simulink model "untitled"  (R2014a)
settings: Solver=ode45  StartTime=0.0  StopTime=10.0  RelTol=1e-3
undefined symbols (not defined in the file or in its folder): sigbuilder_block
libraries: simulink x4
settings Model: Creator=Dell  LastModifiedBy=Dell

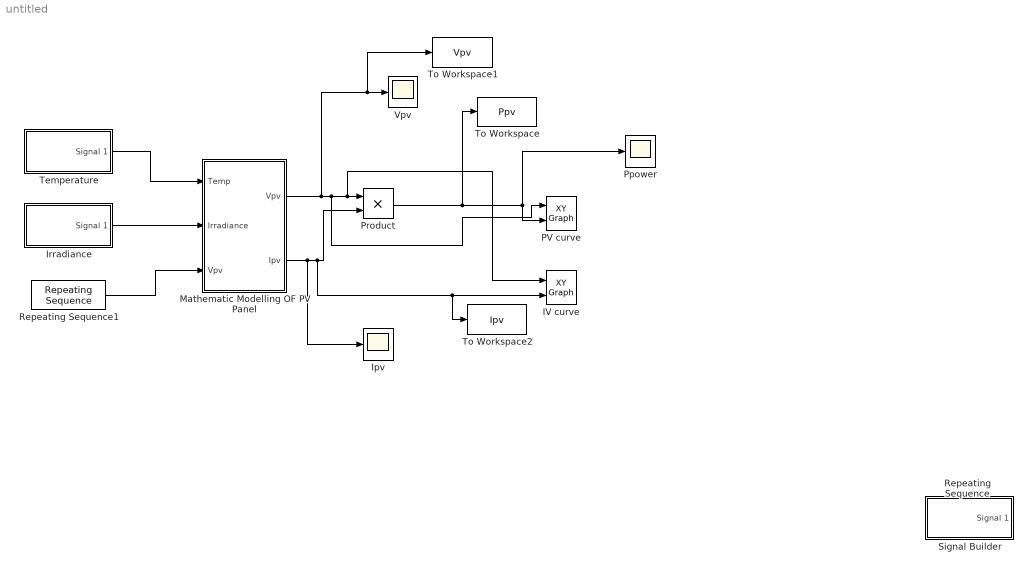
== system untitled ==
  IV curve : simulink/Sinks/XY Graph  xmin=-1  xmax=1  ymin=-1  ymax=1  st=-1
  Ipv : Scope
  Irradiance : Subsystem  Tag=STV Subsys  LoadFcn=sigbuilder_block('load');  StartFcn=sigbuilder_block('start');  StopFcn=sigbuilder_block('stop');  ClipboardFcn=sigbuilder_block('clipboard');  mask(Sigbuilder block){}
      mask help: Simulink:masks:SigbuilderBlock_MD
      mask init:
      | if ~strcmp(get_param(bdroot(gcbh),'SimulationStatus'),'stopped') tuvar = sigbuilder_block('maskInit'); end
      settings: CopyFcn=sigbuilder_block('copy');  DeleteFcn=sigbuilder_block('delete');  ModelCloseFcn=sigbuilder_block('modelClose');  PreSaveFcn=sigbuilder_block('preSave');  PauseFcn=sigbuilder_block('pause');  ContinueFcn=sigbuilder_block('continue');  NameChangeFcn=sigbuilder_block('namechange');  OpenFcn=sigbuilder_block('open',[441 189.75 543 385.5 ]);  CloseFcn=sigbuilder_block('close');
      mask Display: plot(0, 0, 100, 100,[2, 2, 32, 32, 2], [68, 8, 8, 68, 68],[32, 2], [38, 38], [32, 19, 2],[53, 60, 44], [32, 17, 17, 2],[16, 16, 31, 31]);txt = getActiveGroup(gcbh);text(2, 100, txt,'verticalAlignment', 'top');
  Mathematic Modelling OF PV Panel : Subsystem
  PV curve : simulink/Sinks/XY Graph  xmin=-1  xmax=1  ymin=-1  ymax=1  st=-1
  "Ppower " : Scope
      settings: SaveName=ScopeData2
  Product : Product
  Repeating Sequence : simulink/Sources/Repeating Sequence  rep_seq_t=[0 2]  rep_seq_y=[0 2]
  Repeating Sequence1 : simulink/Sources/Repeating Sequence  rep_seq_t=[0 2]  rep_seq_y=[0 2]
  Signal Builder : Subsystem  Tag=STV Subsys  LoadFcn=sigbuilder_block('load');  StartFcn=sigbuilder_block('start');  StopFcn=sigbuilder_block('stop');  ClipboardFcn=sigbuilder_block('clipboard');  mask(Sigbuilder block){}
      mask help: Simulink:masks:SigbuilderBlock_MD
      mask init:
      | if ~strcmp(get_param(bdroot(gcbh),'SimulationStatus'),'stopped') tuvar = sigbuilder_block('maskInit'); end
      settings: CopyFcn=sigbuilder_block('copy');  DeleteFcn=sigbuilder_block('delete');  ModelCloseFcn=sigbuilder_block('modelClose');  PreSaveFcn=sigbuilder_block('preSave');  PauseFcn=sigbuilder_block('pause');  ContinueFcn=sigbuilder_block('continue');  NameChangeFcn=sigbuilder_block('namechange');  OpenFcn=sigbuilder_block('open',[437.6 199.2 550.4 400 ]);  CloseFcn=sigbuilder_block('close');
      mask Display: plot(0, 0, 100, 100,[2, 2, 32, 32, 2], [68, 8, 8, 68, 68],[32, 2], [38, 38], [32, 19, 2],[53, 60, 44], [32, 17, 17, 2],[16, 16, 31, 31]);txt = getActiveGroup(gcbh);text(2, 100, txt,'verticalAlignment', 'top');
  "Temperature " : Subsystem  Tag=STV Subsys  LoadFcn=sigbuilder_block('load');  StartFcn=sigbuilder_block('start');  StopFcn=sigbuilder_block('stop');  ClipboardFcn=sigbuilder_block('clipboard');  mask(Sigbuilder block){}
      mask help: Simulink:masks:SigbuilderBlock_MD
      mask init:
      | if ~strcmp(get_param(bdroot(gcbh),'SimulationStatus'),'stopped') tuvar = sigbuilder_block('maskInit'); end
      settings: CopyFcn=sigbuilder_block('copy');  DeleteFcn=sigbuilder_block('delete');  ModelCloseFcn=sigbuilder_block('modelClose');  PreSaveFcn=sigbuilder_block('preSave');  PauseFcn=sigbuilder_block('pause');  ContinueFcn=sigbuilder_block('continue');  NameChangeFcn=sigbuilder_block('namechange');  OpenFcn=sigbuilder_block('open',[351 -51.75 543 385.5 ]);  CloseFcn=sigbuilder_block('close');
      mask Display: plot(0, 0, 100, 100,[2, 2, 32, 32, 2], [68, 8, 8, 68, 68],[32, 2], [38, 38], [32, 19, 2],[53, 60, 44], [32, 17, 17, 2],[16, 16, 31, 31]);txt = getActiveGroup(gcbh);text(2, 100, txt,'verticalAlignment', 'top');
  To Workspace : ToWorkspace  VariableName=Ppv  SaveFormat=Timeseries  SampleTime=-1
  To Workspace1 : ToWorkspace  VariableName=Vpv  SaveFormat=Timeseries  SampleTime=-1
  To Workspace2 : ToWorkspace  VariableName=Ipv  SaveFormat=Timeseries  SampleTime=-1
  Vpv : Scope
  wires:
  Mathematic Modelling OF PV Panel/2(Ipv) -> Ipv/1, To Workspace2/1, IV curve/2, Product/2
  Mathematic Modelling OF PV Panel/1("Vpv ") -> To Workspace1/1, Vpv/1, PV curve/1, IV curve/1, Product/1
  Product/1 -> To Workspace/1, PV curve/2, "Ppower "/1
  "Temperature "/1(Signal 1) -> Mathematic Modelling OF PV Panel/1(Temp)
  Irradiance/1(Signal 1) -> Mathematic Modelling OF PV Panel/2(Irradiance)
  Repeating Sequence1/1 -> Mathematic Modelling OF PV Panel/3(Vpv)

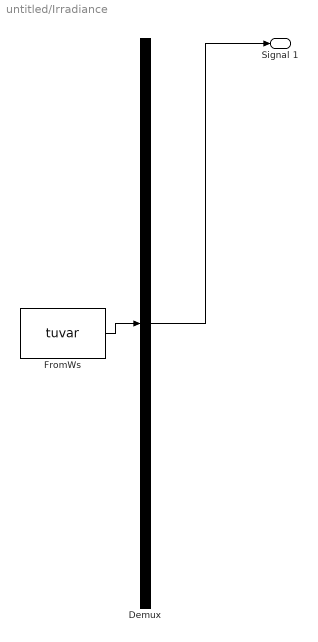
== system untitled/Irradiance ==
  Demux : Demux  Tag=STV Demux  Outputs=1
  FromWs : FromWorkspace  Tag=STV FromWs  VariableName=tuvar  SampleTime=0
      SigBuilderData=|
      | common.afterFinalStr = 'Extrapolate'
      | common.sampleTime = 0
      | dataSet.timeRange = [0 10]
      | dataSet.name = 'Group 1'
      | sbobj.Groups.Name = 'Group 1'
      | sbobj.Groups.Signals.Name = 'Signal 1'
      | sbobj.Groups.Signals.XData = [0 4 4 6 6 10]
      | sbobj.Groups.Signals.YData = [0 0 1 1 0 0]
  Signal 1 : Outport  Tag=STV Outport
  wires:
  Demux/1 -> Signal 1/1
  FromWs/1 -> Demux/1

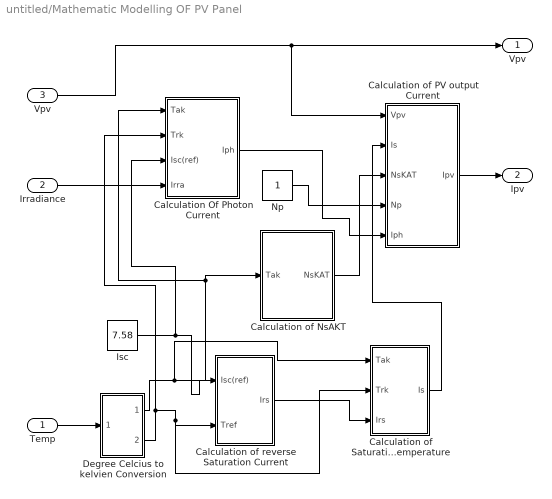
== system untitled/Mathematic Modelling OF PV Panel ==
  Temp : Inport
  Irradiance : Inport  Port=2
  Vpv : Inport  Port=3
  "Calculation Of Photon Current " : Subsystem
  Calculation of Saturation Current Varies With Temperature : Subsystem
  Calculation of NsAKT : Subsystem
  "Calculation of PV output Current " : Subsystem
  Calculation of reverse Saturation Current : Subsystem
  Degree Celcius to kelvien Conversion : Subsystem
  Isc : Constant  Value=7.58
  Np : Constant
  "Vpv " : Outport
  Ipv : Outport  Port=2
  wires:
  Calculation of Saturation Current Varies With Temperature/1(Is) -> "Calculation of PV output Current "/2(Is)
  Calculation of reverse Saturation Current/1(Irs) -> Calculation of Saturation Current Varies With Temperature/3("Irs ")
  Np/1 -> "Calculation of PV output Current "/4(Np)
  Temp/1 -> Degree Celcius to kelvien Conversion/1("Top ")
  "Calculation of PV output Current "/1("Ipv ") -> Ipv/1
  Irradiance/1 -> "Calculation Of Photon Current "/4(Irra)
  Degree Celcius to kelvien Conversion/1(Tak) -> Calculation of Saturation Current Varies With Temperature/1(Tak), "Calculation Of Photon Current "/1(Tak), Calculation of NsAKT/1("Tak ")
  "Calculation Of Photon Current "/1(Iph) -> "Calculation of PV output Current "/5(Iph)
  Calculation of NsAKT/1(NsKAT) -> "Calculation of PV output Current "/3(NsKAT)
  Isc/1 -> "Calculation Of Photon Current "/3(Isc(ref)), Calculation of reverse Saturation Current/1("Isc(ref) ")
  Degree Celcius to kelvien Conversion/2(Trk) -> "Calculation Of Photon Current "/2(Trk), Calculation of Saturation Current Varies With Temperature/2("Trk "), Calculation of reverse Saturation Current/2("Tref ")
  Vpv/1 -> "Vpv "/1, "Calculation of PV output Current "/1(Vpv)

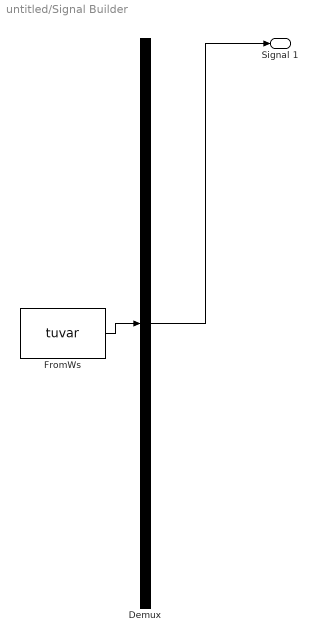
== system untitled/Signal Builder ==
  Demux : Demux  Tag=STV Demux  Outputs=1
  FromWs : FromWorkspace  Tag=STV FromWs  VariableName=tuvar  SampleTime=0
      SigBuilderData=|
      | common.afterFinalStr = 'Extrapolate'
      | common.sampleTime = 0
      | dataSet.timeRange = [0 10]
      | dataSet.name = 'Group 1'
      | sbobj.Groups.Name = 'Group 1'
      | sbobj.Groups.Signals.Name = 'Signal 1'
      | sbobj.Groups.Signals.XData = [0 4 4 6 6 10]
      | sbobj.Groups.Signals.YData = [0 0 1 1 0 0]
  Signal 1 : Outport  Tag=STV Outport
  wires:
  Demux/1 -> Signal 1/1
  FromWs/1 -> Demux/1

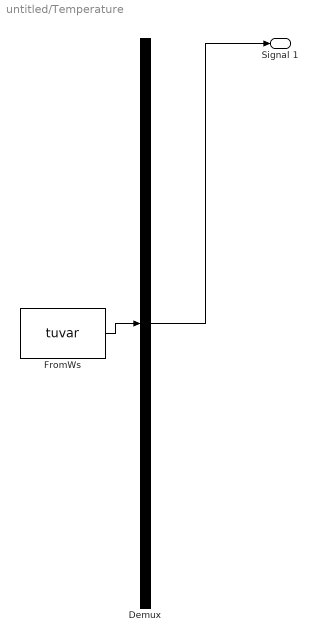
== system untitled/Temperature  ==
  Demux : Demux  Tag=STV Demux  Outputs=1
  FromWs : FromWorkspace  Tag=STV FromWs  VariableName=tuvar  SampleTime=0
      SigBuilderData=|
      | common.afterFinalStr = 'Extrapolate'
      | common.sampleTime = 0
      | dataSet.timeRange = [0 10]
      | dataSet.name = 'Group 1'
      | sbobj.Groups.Name = 'Group 1'
      | sbobj.Groups.Signals.Name = 'Signal 1'
      | sbobj.Groups.Signals.XData = [0 1 1 2 2 10]
      | sbobj.Groups.Signals.YData = [25 25 50 50 75 75]
  Signal 1 : Outport  Tag=STV Outport
  wires:
  FromWs/1 -> Demux/1
  Demux/1 -> Signal 1/1

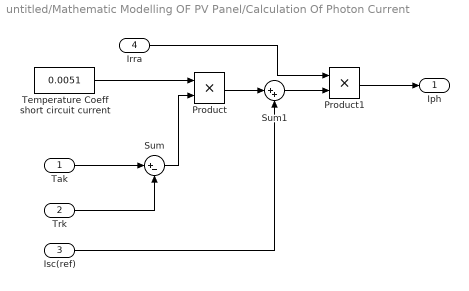
== system untitled/Mathematic Modelling OF PV Panel/Calculation Of Photon Current  ==
  Tak : Inport
  Trk : Inport  Port=2
  Isc(ref) : Inport  Port=3
  Irra : Inport  Port=4
  Product : Product
  Product1 : Product
  Sum : Sum  Inputs=|+-
  Sum1 : Sum  Inputs=|++
  "Temperature Coeff short circuit current " : Constant  Value=0.0051
  Iph : Outport
  wires:
  Product/1 -> Sum1/1
  Trk/1 -> Sum/2
  "Temperature Coeff short circuit current "/1 -> Product/1
  Irra/1 -> Product1/1
  Isc(ref)/1 -> Sum1/2
  Tak/1 -> Sum/1
  Sum1/1 -> Product1/2
  Sum/1 -> Product/2
  Product1/1 -> Iph/1

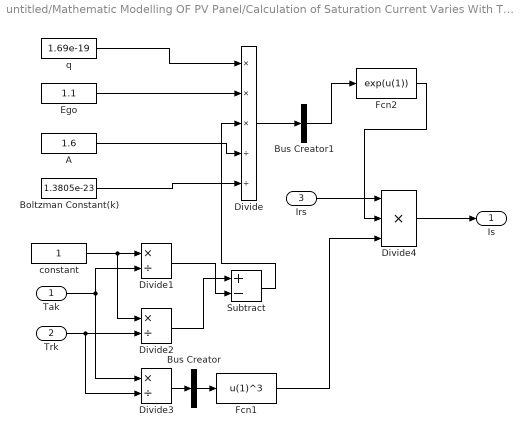
== system untitled/Mathematic Modelling OF PV Panel/Calculation of Saturation Current Varies With Temperature ==
  Tak : Inport
  "Trk " : Inport  Port=2
  "Irs " : Inport  Port=3
  "A " : Constant  Value=1.6
  Boltzman Constant(k) : Constant  Value=1.3805e-23
  Bus Creator : BusCreator  Inputs=1
  Bus Creator1 : BusCreator  Inputs=1
  Divide : Product  Inputs=***//
  Divide1 : Product  Inputs=*/
  Divide2 : Product  Inputs=*/
  Divide3 : Product  Inputs=*/
  Divide4 : Product  Inputs=***
  Ego : Constant  Value=1.1
  Fcn1 : Fcn  Expr=u(1)^3
  Fcn2 : Fcn  Expr=exp(u(1))
  Subtract : Sum  Inputs=+-
  "constant " : Constant
  "q " : Constant  Value=1.69e-19
  Is : Outport
  wires:
  "constant "/1 -> Divide2/1, Divide1/1
  Bus Creator1/1 -> Fcn2/1
  Divide/1 -> Bus Creator1/1
  Divide1/1 -> Subtract/2
  Fcn1/1 -> Divide4/3
  Divide2/1 -> Subtract/1
  Tak/1 -> Divide1/2, Divide3/1
  Fcn2/1 -> Divide4/2
  "Trk "/1 -> Divide3/2, Divide2/2
  "A "/1 -> Divide/4
  Ego/1 -> Divide/2
  Subtract/1 -> Divide/3
  Boltzman Constant(k)/1 -> Divide/5
  "q "/1 -> Divide/1
  "Irs "/1 -> Divide4/1
  Divide4/1 -> Is/1
  Bus Creator/1 -> Fcn1/1
  Divide3/1 -> Bus Creator/1

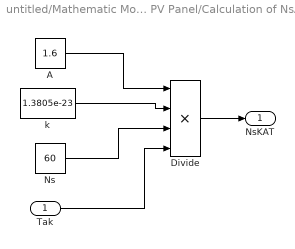
== system untitled/Mathematic Modelling OF PV Panel/Calculation of NsAKT ==
  "Tak " : Inport
  A : Constant  Value=1.6
  Divide : Product  Inputs=****
  Ns : Constant  Value=60
  k : Constant  Value=1.3805e-23
  NsKAT : Outport
  wires:
  Ns/1 -> Divide/3
  A/1 -> Divide/1
  k/1 -> Divide/2
  "Tak "/1 -> Divide/4
  Divide/1 -> NsKAT/1

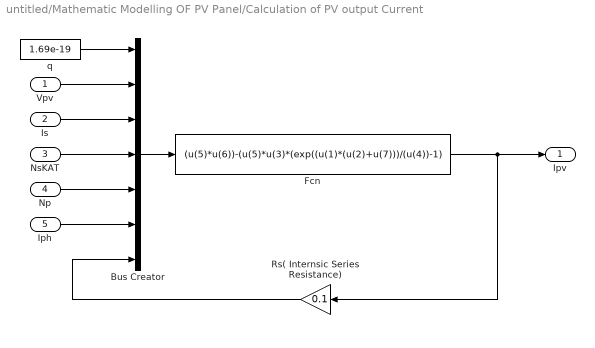
== system untitled/Mathematic Modelling OF PV Panel/Calculation of PV output Current  ==
  Vpv : Inport
  Is : Inport  Port=2
  NsKAT : Inport  Port=3
  Np : Inport  Port=4
  Iph : Inport  Port=5
  Bus Creator : BusCreator  Inputs=7
  Fcn : Fcn  Expr=(u(5)*u(6))-(u(5)*u(3)*(exp((u(1)*(u(2)+u(7)))/(u(4))-1)
  Rs( Internsic Series Resistance) : Gain  Gain=0.1
  q : Constant  Value=1.69e-19
  "Ipv " : Outport
  wires:
  Vpv/1 -> Bus Creator/2
  Is/1 -> Bus Creator/3
  Fcn/1 -> "Ipv "/1, Rs( Internsic Series Resistance)/1
  Bus Creator/1 -> Fcn/1
  Rs( Internsic Series Resistance)/1 -> Bus Creator/7
  Iph/1 -> Bus Creator/6
  Np/1 -> Bus Creator/5
  q/1 -> Bus Creator/1
  NsKAT/1 -> Bus Creator/4

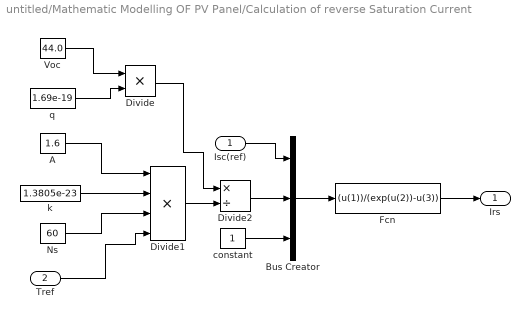
== system untitled/Mathematic Modelling OF PV Panel/Calculation of reverse Saturation Current ==
  "Isc(ref) " : Inport
  "Tref " : Inport  Port=2
  A : Constant  Value=1.6
  Bus Creator : BusCreator  Inputs=3
  Divide : Product  Inputs=**
  Divide1 : Product  Inputs=****
  Divide2 : Product  Inputs=*/
  Fcn : Fcn  Expr=(u(1))/(exp(u(2))-u(3))
  Ns : Constant  Value=60
  Voc : Constant  Value=44.0
  "constant " : Constant
  k : Constant  Value=1.3805e-23
  q : Constant  Value=1.69e-19
  Irs : Outport
  wires:
  Voc/1 -> Divide/1
  Divide/1 -> Divide2/1
  k/1 -> Divide1/2
  "constant "/1 -> Bus Creator/3
  Divide2/1 -> Bus Creator/2
  Bus Creator/1 -> Fcn/1
  "Tref "/1 -> Divide1/4
  Fcn/1 -> Irs/1
  q/1 -> Divide/2
  A/1 -> Divide1/1
  "Isc(ref) "/1 -> Bus Creator/1
  Ns/1 -> Divide1/3
  Divide1/1 -> Divide2/2

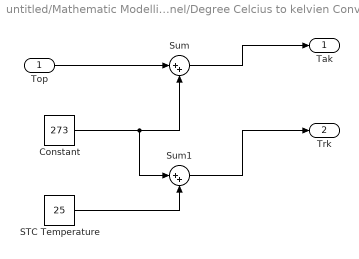
== system untitled/Mathematic Modelling OF PV Panel/Degree Celcius to kelvien Conversion ==
  "Top " : Inport
  Constant : Constant  Value=273
  STC Temperature : Constant  Value=25
  Sum : Sum  Inputs=|++
  Sum1 : Sum  Inputs=|++
  Tak : Outport
  Trk : Outport  Port=2
  wires:
  Sum1/1 -> Trk/1
  Constant/1 -> Sum1/1, Sum/2
  "Top "/1 -> Sum/1
  Sum/1 -> Tak/1
  STC Temperature/1 -> Sum1/2
